simulink model "logging_task"  (Simulink 3.00)
libraries: genlib x4, mathlib x2, timelib x2, logiclib x2, speclib x1, analoglib x1

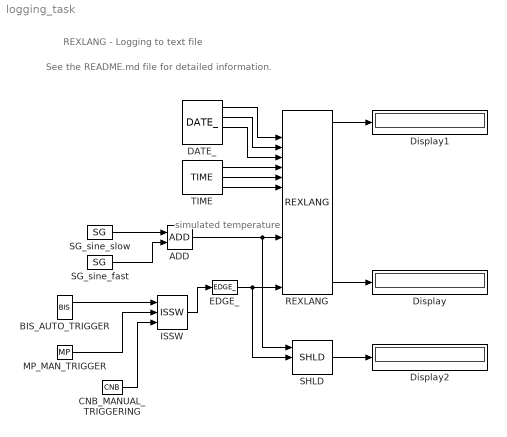
== system logging_task ==
  note: See the README.md file for detailed information.
  note: REXLANG - Logging to text file
  note: simulated
      | temperature
  ADD : mathlib/ADD
  BIS_AUTO_TRIGGER : genlib/BIS  Y0=on  t1=30  t2=60  t3=0  t4=4  t5=5  t6=6  t7=7  t8=8  RPT=on
  CNB_MANUAL_TRIGGERING : mathlib/CNB  YCN=off
  DATE_ : timelib/DATE_  tz=1: Local time
  Display : Display
      settings: Format=Best fit  Suffix=chars
  Display1 : Display
      settings: Format=Best fit
  Display2 : Display
      settings: Format=short  Suffix=°C
  EDGE_ : logiclib/EDGE_  iedge=1: Rising edge
  ISSW : logiclib/ISSW
  MP_MAN_TRIGGER : genlib/MP  BSTATE=on  pwidth=1  RPTF=off
  REXLANG : speclib/REXLANG  strs=0  SystemSampleTime=-1  tab_matlab=BASIC  srcname=logging_rexlang.c  srctype=1: C-like  stack=0  debug=3: Full check  p0=0  p1=0  p2=0  p3=0  p4=0  p5=0  p6=0  p7=0  p8=0  p9=0  p10=0  p11=0  p12=0  p13=0  p14=0  p15=0
  SG_sine_fast : genlib/SG  isig=1: SINE  amp=3  freq=0.09  phase=0  ifrunit=1: Hz  iphunit=1: degrees  offset=0
  SG_sine_slow : genlib/SG  isig=1: SINE  amp=10  freq=0.025  phase=0  ifrunit=1: Hz  iphunit=1: degrees  offset=5
  SHLD : analoglib/SHLD  y0=0  mode=1: Triggered sampling
  TIME : timelib/TIME  tz=1: Local time
  wires:
  ADD/1 -> REXLANG/13, SHLD/1
  BIS_AUTO_TRIGGER/1 -> ISSW/1
  CNB_MANUAL_TRIGGERING/1 -> ISSW/3
  DATE_/1 -> REXLANG/3
  DATE_/2 -> REXLANG/4
  DATE_/3 -> REXLANG/5
  EDGE_/1 -> REXLANG/18, SHLD/2
  ISSW/1 -> EDGE_/1
  MP_MAN_TRIGGER/1 -> ISSW/2
  REXLANG/1 -> Display1/1
  REXLANG/17 -> Display/1
  SG_sine_fast/1 -> ADD/2
  SG_sine_slow/1 -> ADD/1
  SHLD/1 -> Display2/1
  TIME/1 -> REXLANG/6
  TIME/2 -> REXLANG/7
  TIME/3 -> REXLANG/8
